simulink model "setupModel"  (R2025b)
settings: Solver=VariableStepAuto  StartTime=0.0  StopTime=10.0  RelTol=1e-3
undefined symbols (not defined in the file or in its folder): DiscIntNeverNeededParam
settings Model: Creator=sung0058  LastModifiedBy=sung0058

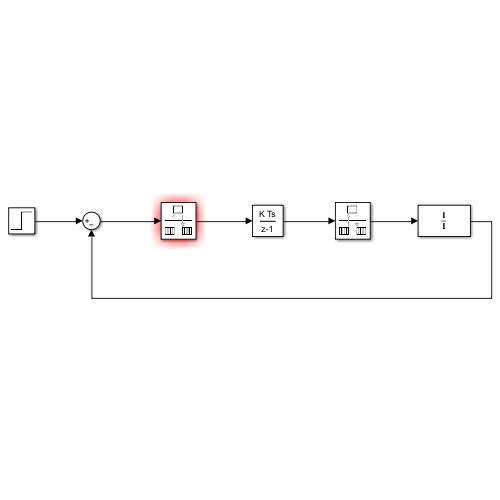
[thumbnail: Simulink's stored preview of the top-level diagram]
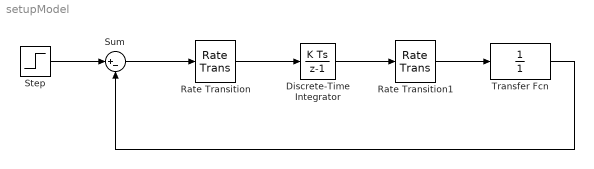
== system setupModel ==
  Discrete-Time Integrator : DiscreteIntegrator  SampleTime=-1  ICPrevOutput=DiscIntNeverNeededParam  ICPrevScaledInput=DiscIntNeverNeededParam
  Rate Transition : RateTransition  OutPortSampleTime=Ts
  Rate Transition1 : RateTransition
  Step : Step  SampleTime=0
  Sum : Sum  Inputs=|+-
  Transfer Fcn : TransferFcn  Denominator=[1]
  wires:
  Sum/1 -> Rate Transition/1
  Discrete-Time Integrator/1 -> Rate Transition1/1
  Step/1 -> Sum/1
  Transfer Fcn/1 -> Sum/2
  Rate Transition/1 -> Discrete-Time Integrator/1
  Rate Transition1/1 -> Transfer Fcn/1
